simulink model "sampleModel1447"  (R2023a)
settings: Solver=VariableStepAuto  StartTime=0.0  StopTime=10.0  RelTol=1e-3
libraries: hdlsllib x7, simulink x4
settings Model: Creator=user1  LastModifiedBy=user1

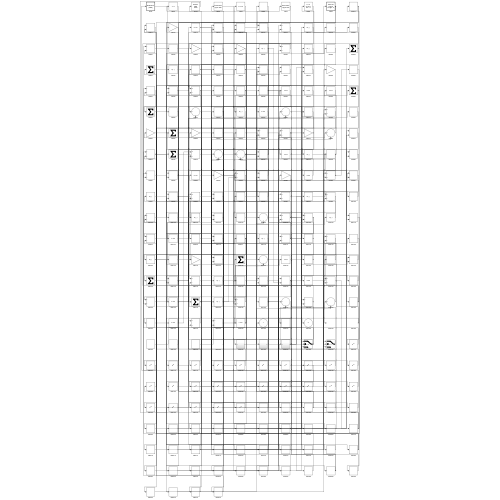
[thumbnail: Simulink's stored preview of the top-level diagram]
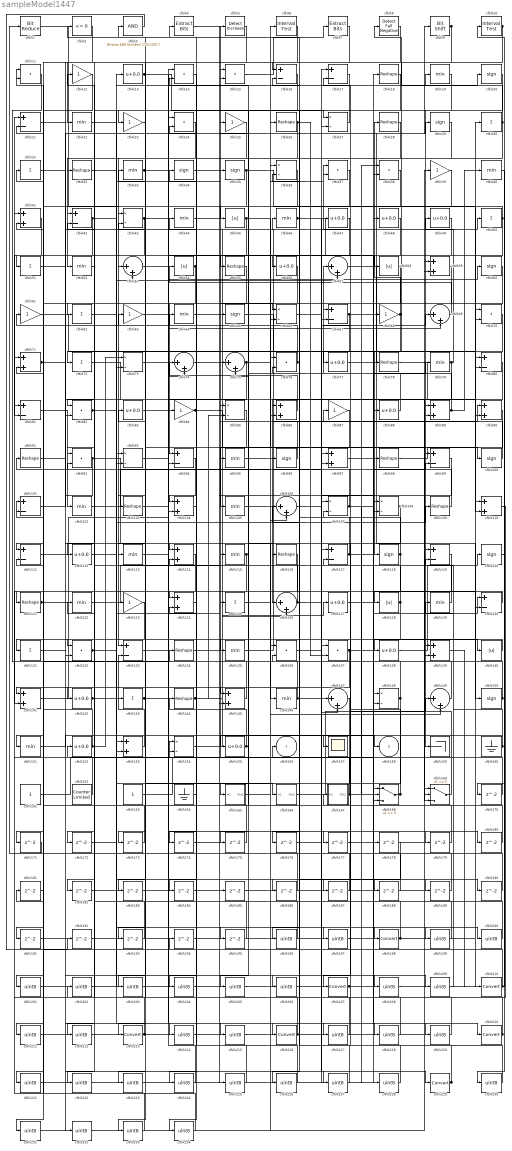
== system sampleModel1447 ==
  cfblk1 : hdlsllib/Logic and Bit Operations/Bit Reduce  mode=AND
  cfblk10 : hdlsllib/Logic and Bit Operations/Interval Test  IntervalClosedRight=on  uplimit=0.5  IntervalClosedLeft=on  lowlimit=-0.5  OutDataTypeStr=boolean
  cfblk{20,29,34..35,60,65,96,100,118,120,150} (11 alike) : Signum
  cfblk{16..17,21,42,67,80..81,94,99,101,111,117,119,130,133} (15 alike) : Sum  Inputs=+-
  cfblk{19,22,33,40,44,46,52,64,79,95,102,105,113,115,122,129,135,146,151} (19 alike) : MinMax
  cfblk{18,26,28,32,55,78,91,98,103,109,116,121,134,144} (14 alike) : Reshape
  cfblk{41,59,71,86,89..90,97,104,110,114,124,139,141,145,153} (15 alike) : Sum
  cfblk{53,57,69,74..75,106,126,147,149} (9 alike) : Sum  Inputs=|++
  cfblk{27,36,43,66,73,85,93,107..108,148,154} (11 alike) : Product  Inputs=*/  RndMeth=Zero  SaturateOnIntegerOverflow=on
  cfblk{11,14..15,24,37..38,70,76,82,92,132,136..137} (13 alike) : DotProduct  OutDataTypeStr=Inherit: Inherit via internal rule
  cfblk{13,47..49,56,77,83,88,112,127,138,142,152,155} (14 alike) : Bias  Bias=0.0  SaturateOnIntegerOverflow=off
  cfblk{12,23,25,39,61,63,68,84,87,123} (10 alike) : Gain
  cfblk{30..31,50..51,62,72,125,131,143} (9 alike) : Sum  Inputs=+
  cfblk{45,54,58,128,140} (5 alike) : Abs  SaturateOnIntegerOverflow=off
  cfblk157 : Scope
  cfblk159 : Terminator
  cfblk160 : Ground
  cfblk161 : Constant  SampleTime=-1
  cfblk162 : hdlsllib/Sources/Counter Limited  uplimit=7  tsamp=-1
  cfblk163 : Constant  SampleTime=-1
  cfblk164 : Ground
  cfblk165 : Subsystem
      settings: LibrarySourceBlock=|
      | hdlsllib/Ports &
      | Subsystems/Subsystem
  cfblk166 : Subsystem
      settings: LibrarySourceBlock=|
      | hdlsllib/Ports &
      | Subsystems/Subsystem
  cfblk167 : Subsystem
      settings: LibrarySourceBlock=|
      | hdlsllib/Ports &
      | Subsystems/Subsystem
  cfblk168 : Switch  SaturateOnIntegerOverflow=off  InputSameDT=off
  cfblk169 : Switch  SaturateOnIntegerOverflow=off  InputSameDT=off
  cfblk{170..195} (26 alike) : Delay  SampleTime=1
  cfblk{196..197,199..206,208..209,211..212,214..215,217..219,221..228,230..234} (32 alike) : DataTypeConversion  OutDataTypeStr=uint8  SaturateOnIntegerOverflow=off  RndMeth=Floor
  cfblk{198,207,210,213,216,220,229} (7 alike) : DataTypeConversion  SaturateOnIntegerOverflow=off  RndMeth=Floor
  cfblk2 : hdlsllib/Logic and Bit Operations/Compare To Zero  relop=<=  OutDataTypeStr=boolean
  cfblk3 : simulink/Logic and Bit Operations/Bitwise Operator  logicop=AND  UseBitMask=on  BitMask=bin2dec('11011001')  BitMaskRealWorld=Stored Integer
      settings: LibrarySourceBlock=|
      | hdlsllib/Logic and Bit
      | Operations/Bitwise
      | Operator
  cfblk4 : simulink/Logic and Bit Operations/Extract Bits  bitsToExtract=Upper half  numBits=8  bitIdxRange=[0 7]  outScalingMode=Preserve fixed-point scaling
      settings: LibrarySourceBlock=|
      | hdlsllib/Logic and Bit
      | Operations/Extract Bits
  cfblk5 : simulink/Logic and Bit Operations/Detect Increase  vinit=0.0  OutDataTypeStr=boolean
      settings: LibrarySourceBlock=|
      | hdlsllib/Logic and Bit
      | Operations/Detect
      | Increase
  cfblk6 : hdlsllib/Logic and Bit Operations/Interval Test  IntervalClosedRight=on  uplimit=0.5  IntervalClosedLeft=on  lowlimit=-0.5  OutDataTypeStr=boolean
  cfblk7 : simulink/Logic and Bit Operations/Extract Bits  bitsToExtract=Upper half  numBits=8  bitIdxRange=[0 7]  outScalingMode=Preserve fixed-point scaling
      settings: LibrarySourceBlock=|
      | hdlsllib/Logic and Bit
      | Operations/Extract Bits
  cfblk8 : hdlsllib/Logic and Bit Operations/Detect Fall Negative  vinit=0  OutDataTypeStr=boolean
  cfblk9 : hdlsllib/Logic and Bit Operations/Bit Shift  mode=Shift Left Logical  N=0
  cfblk156 : Outport  VectorParamsAs1DForOutWhenUnconnected=off
  cfblk158 : Outport  Port=2  VectorParamsAs1DForOutWhenUnconnected=off
  wires:
  cfblk163/1 -> cfblk5/1
  cfblk76/1 -> cfblk61/1, cfblk36/2
  cfblk26/1 -> cfblk133/1, cfblk137/2
  cfblk20/1 -> cfblk159/1
  cfblk118/1 -> cfblk91/1, cfblk132/1
  cfblk11/1 -> cfblk134/1
  cfblk94/1 -> cfblk104/1
  cfblk98/1 -> cfblk100/1
  cfblk139/1 -> cfblk210/1
  cfblk54/1 -> cfblk94/1, cfblk174/1
  cfblk124/1 -> cfblk64/1
  cfblk70/1 -> cfblk72/1
  cfblk146/1 -> cfblk69/1, cfblk44/1, cfblk189/1
  cfblk27/1 -> cfblk23/1
  cfblk86/1 -> cfblk74/1
  cfblk8/1 -> cfblk113/1
  cfblk154/1 -> cfblk46/1
  cfblk29/1 -> cfblk52/1
  cfblk143/1 -> cfblk43/2, cfblk200/1, cfblk206/1
  cfblk138/1 -> cfblk120/1
  cfblk61/1 -> cfblk118/1
  cfblk81/1 -> cfblk102/1
  cfblk101/1 -> cfblk50/1
  cfblk58/1 -> cfblk131/1
  cfblk114/1 -> cfblk121/1
  cfblk148/1 -> cfblk101/1, cfblk233/1
  cfblk111/1 -> cfblk114/1
  cfblk96/1 -> cfblk65/1
  cfblk132/1 -> cfblk125/1, cfblk35/1
  cfblk74/1 -> cfblk75/1
  cfblk68/1 -> cfblk28/1, cfblk184/1
  cfblk153/1 -> cfblk133/2
  cfblk135/1 -> cfblk90/1
  cfblk95/1 -> cfblk37/1
  cfblk121/1 -> cfblk73/2, cfblk217/1
  cfblk166/1(Out1) -> cfblk149/1
  cfblk30/1 -> cfblk124/1, cfblk8/1
  cfblk80/1 -> cfblk126/1
  cfblk112/1 -> cfblk19/1
  cfblk77/1 -> cfblk9/1
  cfblk147/1 -> cfblk213/1
  cfblk43/1 -> cfblk81/2, cfblk215/1
  cfblk88/1 -> cfblk57/1
  cfblk50/1 -> cfblk45/1, cfblk103/1
  cfblk155/1 -> cfblk75/2, cfblk4/1
  cfblk144/1 -> cfblk127/1, cfblk85/2
  cfblk51/1 -> cfblk29/1
  cfblk141/1 -> cfblk94/2
  cfblk85/1 -> cfblk105/1
  cfblk44/1 -> cfblk96/1
  cfblk42/1 -> cfblk13/1, cfblk211/1
  cfblk15/1 -> cfblk7/1
  cfblk93/1 -> cfblk60/1
  cfblk122/1 -> cfblk115/1
  cfblk134/1 -> cfblk126/2
  cfblk151/1 -> cfblk158/1
  cfblk130/1 -> cfblk128/1
  cfblk52/1 -> cfblk142/1
  cfblk97/1 -> cfblk220/1
  cfblk125/1 -> cfblk6/1
  cfblk4/1 -> cfblk66/1
  cfblk160/1 -> cfblk129/1, cfblk155/1
  cfblk65/1 -> cfblk77/1
  cfblk145/1 -> cfblk34/1
  cfblk92/1 -> cfblk146/1, cfblk132/2, cfblk190/1, cfblk212/1
  cfblk36/1 -> cfblk141/1
  cfblk115/1 -> cfblk145/1, cfblk141/2
  cfblk32/1 -> cfblk143/1
  cfblk56/1 -> cfblk135/1
  cfblk168/1 -> cfblk67/1, cfblk154/1
  cfblk1/1 -> cfblk43/1
  cfblk57/1 -> cfblk150/1
  cfblk22/1 -> cfblk166/1(In1)
  cfblk62/1 -> cfblk57/2
  cfblk13/1 -> cfblk27/1, cfblk58/1
  cfblk82/1 -> cfblk88/1, cfblk199/1
  cfblk105/1 -> cfblk67/2
  cfblk41/1 -> cfblk51/1
  cfblk75/1 -> cfblk26/1, cfblk37/2, cfblk104/2, cfblk99/1
  cfblk150/1 -> cfblk85/1, cfblk25/1
  cfblk142/1 -> cfblk93/2, cfblk109/1
  cfblk152/1 -> cfblk41/2, cfblk73/1
  cfblk59/1 -> cfblk92/1
  cfblk84/1 -> cfblk169/3, cfblk208/1
  cfblk2/1 -> cfblk22/1
  cfblk69/1 -> cfblk54/1
  cfblk136/1 -> cfblk198/1
  cfblk53/1 -> cfblk86/1
  cfblk169/1 -> cfblk95/1
  cfblk161/1 -> cfblk148/1
  cfblk33/1 -> cfblk186/1, cfblk187/1
  cfblk129/1 -> cfblk92/2
  cfblk45/1 -> cfblk90/2, cfblk55/1
  cfblk119/1 -> cfblk207/1
  cfblk108/1 -> cfblk157/1, cfblk175/1
  cfblk149/1 -> cfblk12/1
  cfblk55/1 -> cfblk111/1
  cfblk5/1 -> cfblk32/1
  cfblk37/1 -> cfblk56/1
  cfblk106/1 -> cfblk229/1
  cfblk9/1 -> cfblk82/1, cfblk82/2
  cfblk28/1 -> cfblk62/1
  cfblk79/1 -> cfblk169/2, cfblk49/1
  cfblk47/1 -> cfblk84/1
  cfblk71/1 -> cfblk116/1, cfblk89/2
  cfblk126/1 -> cfblk33/1, cfblk188/1
  cfblk6/1 -> cfblk16/1
  cfblk128/1 -> cfblk3/1, cfblk193/1
  cfblk78/1 -> cfblk110/1
  cfblk66/1 -> cfblk108/1
  cfblk38/1 -> cfblk151/1
  cfblk162/1 -> cfblk11/1
  cfblk35/1 -> cfblk110/2, cfblk182/1
  cfblk117/1 -> cfblk140/1, cfblk107/2, cfblk2/1, cfblk99/2
  cfblk16/1 -> cfblk165/1(In1)
  cfblk67/1 -> cfblk18/1, cfblk112/1
  cfblk99/1 -> cfblk145/2
  cfblk102/1 -> cfblk66/2
  cfblk23/1 -> cfblk53/1
  cfblk133/1 -> cfblk69/2
  cfblk107/1 -> cfblk71/2, cfblk130/2, cfblk79/1, cfblk228/1
  cfblk10/1 -> cfblk78/1, cfblk191/1
  cfblk19/1 -> cfblk153/2
  cfblk46/1 -> cfblk148/2, cfblk80/2
  cfblk140/1 -> cfblk138/1
  cfblk89/1 -> cfblk14/2, cfblk40/1
  cfblk167/1(Out1) -> cfblk156/1, cfblk98/1, cfblk38/1, cfblk20/1
  cfblk31/1 -> cfblk216/1
  cfblk7/1 -> cfblk42/1
  cfblk109/1 -> cfblk47/1
  cfblk164/1 -> cfblk124/2
  cfblk100/1 -> cfblk15/1
  cfblk137/1 -> cfblk130/1, cfblk231/1
  cfblk72/1 -> cfblk117/1
  cfblk165/1(Out1) -> cfblk149/2
  cfblk120/1 -> cfblk170/1
  cfblk170/1 -> cfblk41/1
  cfblk116/1 -> cfblk171/1
  cfblk171/1 -> cfblk1/1
  cfblk18/1 -> cfblk172/1
  cfblk90/1 -> cfblk173/1
  cfblk173/1 -> cfblk153/1
  cfblk175/1 -> cfblk111/2
  cfblk87/1 -> cfblk176/1
  cfblk176/1 -> cfblk27/2
  cfblk64/1 -> cfblk177/1
  cfblk177/1 -> cfblk89/1
  cfblk83/1 -> cfblk179/1
  cfblk179/1 -> cfblk15/2
  cfblk127/1 -> cfblk180/1
  cfblk180/1 -> cfblk93/1
  cfblk181/1 -> cfblk101/2
  cfblk182/1 -> cfblk168/2
  cfblk25/1 -> cfblk183/1
  cfblk183/1 -> cfblk74/2
  cfblk184/1 -> cfblk59/2
  cfblk34/1 -> cfblk185/1
  cfblk185/1 -> cfblk86/2
  cfblk186/1 -> cfblk71/1
  cfblk187/1 -> cfblk137/1
  cfblk188/1 -> cfblk154/2
  cfblk189/1 -> cfblk117/2
  cfblk190/1 -> cfblk114/2
  cfblk191/1 -> cfblk107/1
  cfblk3/1 -> cfblk192/1
  cfblk192/1 -> cfblk53/2
  cfblk193/1 -> cfblk42/2
  cfblk194/1 -> cfblk168/1
  cfblk103/1 -> cfblk195/1
  cfblk195/1 -> cfblk14/1
  cfblk178/1 -> cfblk196/1
  cfblk196/1 -> cfblk76/1
  cfblk113/1 -> cfblk197/1
  cfblk197/1 -> cfblk178/1
  cfblk198/1 -> cfblk80/1, cfblk122/1, cfblk76/2
  cfblk199/1 -> cfblk136/1
  cfblk200/1 -> cfblk136/2
  cfblk123/1 -> cfblk201/1
  cfblk201/1 -> cfblk68/1
  cfblk110/1 -> cfblk202/1
  cfblk202/1 -> cfblk123/1
  cfblk48/1 -> cfblk203/1
  cfblk203/1 -> cfblk70/2
  cfblk60/1 -> cfblk204/1
  cfblk204/1 -> cfblk48/1
  cfblk39/1 -> cfblk205/1
  cfblk205/1 -> cfblk70/1
  cfblk206/1 -> cfblk39/1
  cfblk207/1 -> cfblk38/2, cfblk30/1
  cfblk208/1 -> cfblk119/1
  cfblk91/1 -> cfblk209/1
  cfblk209/1 -> cfblk119/2
  cfblk210/1 -> cfblk11/2, cfblk16/2, cfblk10/1
  cfblk211/1 -> cfblk139/1
  cfblk212/1 -> cfblk139/2
  cfblk213/1 -> cfblk108/2, cfblk152/1
  cfblk172/1 -> cfblk214/1
  cfblk214/1 -> cfblk147/1
  cfblk215/1 -> cfblk147/2
  cfblk216/1 -> cfblk36/1, cfblk81/1
  cfblk217/1 -> cfblk31/1
  cfblk63/1 -> cfblk218/1
  cfblk218/1 -> cfblk167/1(In1)
  cfblk73/1 -> cfblk219/1
  cfblk219/1 -> cfblk63/1
  cfblk220/1 -> cfblk181/1, cfblk144/1, cfblk83/1
  cfblk12/1 -> cfblk221/1
  cfblk221/1 -> cfblk97/1
  cfblk49/1 -> cfblk222/1
  cfblk222/1 -> cfblk97/2
  cfblk24/1 -> cfblk223/1
  cfblk223/1 -> cfblk168/3
  cfblk14/1 -> cfblk224/1
  cfblk224/1 -> cfblk24/1
  cfblk174/1 -> cfblk225/1
  cfblk225/1 -> cfblk24/2
  cfblk17/1 -> cfblk226/1
  cfblk226/1 -> cfblk194/1
  cfblk131/1 -> cfblk227/1
  cfblk227/1 -> cfblk17/1
  cfblk228/1 -> cfblk17/2
  cfblk229/1 -> cfblk59/1, cfblk87/1
  cfblk40/1 -> cfblk230/1
  cfblk230/1 -> cfblk106/1
  cfblk231/1 -> cfblk106/2
  cfblk21/1 -> cfblk232/1
  cfblk232/1 -> cfblk169/1
  cfblk233/1 -> cfblk21/1
  cfblk104/1 -> cfblk234/1
  cfblk234/1 -> cfblk21/2

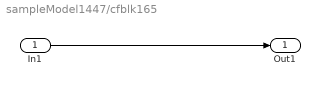
== system sampleModel1447/cfblk165 ==
  In1 : Inport
  Out1 : Outport
  wires:
  In1/1 -> Out1/1

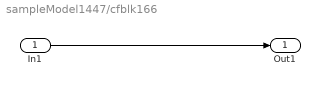
== system sampleModel1447/cfblk166 ==
  In1 : Inport
  Out1 : Outport
  wires:
  In1/1 -> Out1/1

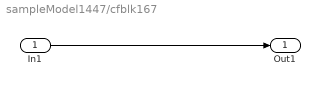
== system sampleModel1447/cfblk167 ==
  In1 : Inport
  Out1 : Outport
  wires:
  In1/1 -> Out1/1
